simulink model "case2_both"  (R2015b)
settings: Solver=FixedStepAuto  StartTime=0.05  StopTime=endtime  FixedStep=0.05  RelTol=1e-3
values from neighbouring files (symbols this model uses):
  AdBottom = (pi*(0.01)^2)/4    (= 7.85398163397e-05)    [case1.m]    (also in case1_val.m; case2.m; case2_val.m; case3.m)
  AdTop = (pi*(0.295*0.0254)^2)/4    (= 4.40962183685e-05)    [case1.m]    (also in case1_val.m; case2.m; case2_val.m; case3.m)
  AreaBottom = (pi*(0.08)^2)/4    (= 0.00502654824574)    [case1.m]    (also in case1_val.m; case2.m; case2_val.m; case3.m)
  AreaTop = (pi*(0.08)^2)/4    (= 0.00502654824574)    [case1.m]    (also in case1_val.m; case2.m; case2_val.m; case3.m)
  Cd1 = b1(i)    [case2.m]    (also in case2_val.m = 0.96)
  Cd2 = b2(i)    [case2.m]    (also in case2_val.m = 0.45)
  g = 9.81    [case1.m]    (also in case1_val.m; case2.m; case2_val.m; case3.m)
  H1_IC = (3.59E+01)*0.01    (= 0.359)    [case2.m]    (also in case2_val.m = 0.177; case3_val.m = 0.177)
  H2_IC = (2.41E+01)*0.01    (= 0.241)    [case2_val.m]    (also in case3_val.m)
settings Model: Creator=guilh_000  LastModifiedBy=guilh_000

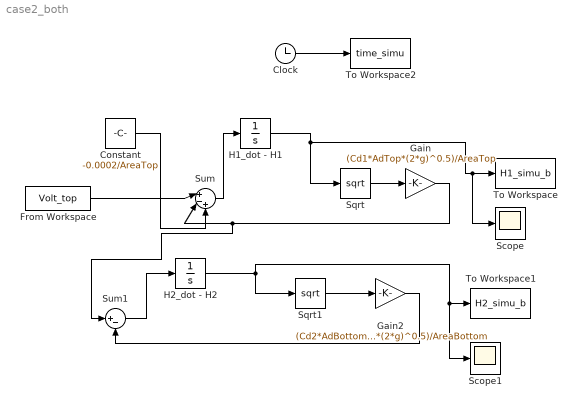
== system case2_both ==
  Clock : Clock
  Constant : Constant  Value=-0.0002/AreaTop
  From Workspace : FromWorkspace  VariableName=Volt_top  SampleTime=0
  Gain : Gain  Gain=(Cd1*AdTop*(2*g)^0.5)/AreaTop
  Gain2 : Gain  Gain=(Cd2*AdBottom*(2*g)^0.5)/AreaBottom
  H1_dot - H1 : Integrator  InitialCondition=H1_IC
  H2_dot - H2 : Integrator  InitialCondition=H2_IC
  Scope : Scope
  Scope1 : Scope
  Sqrt : Sqrt  SaturateOnIntegerOverflow=on
  Sqrt1 : Sqrt  SaturateOnIntegerOverflow=on
  Sum : Sum  Inputs=|+-+
  Sum1 : Sum  Inputs=|+-
  To Workspace : ToWorkspace  VariableName=H1_simu_b  SampleTime=-1
  To Workspace1 : ToWorkspace  VariableName=H2_simu_b  SampleTime=-1
  To Workspace2 : ToWorkspace  VariableName=time_simu  SampleTime=-1
  wires:
  Sum/1 -> H1_dot - H1/1
  Sqrt/1 -> Gain/1
  Gain/1 -> Sum1/1, Sum/2
  From Workspace/1 -> Sum/1
  H2_dot - H2/1 -> Sqrt1/1, Scope1/1, To Workspace1/1
  Sqrt1/1 -> Gain2/1
  Gain2/1 -> Sum1/2
  Sum1/1 -> H2_dot - H2/1
  Clock/1 -> To Workspace2/1
  H1_dot - H1/1 -> Scope/1, To Workspace/1, Sqrt/1
  Constant/1 -> Sum/3
